simulink model "TST_AFST_DD"  (R2016b)
settings: Solver=FixedStepDiscrete  StartTime=0.0  StopTime=simTime  FixedStep=sampleTime  RelTol=1e-3
values from neighbouring files (symbols this model uses):
  testCase = 1    [initTST_AFST_DD_001.m]    (also in initTST_AFST_DD_002.m = 2; initTST_AFST_DD_003.m = 3; initTST_AFST_DD_004.m = 4)
libraries: simulink x61, UnitTest_Lib x56
(part 2 of 2)

== system TST_AFST_DD/simulationInput/testSignals_R004 ==
  BC : BusCreator  Inputs=19
  spec_Air_bDtyCycHiDebTAFS_DSM : FromWorkspace  VariableName=testSig_Air_bDtyCycHiDebTAFS_DSM  Interpolate=off  OutputAfterFinalValue=Holding final value
  spec_Air_bDtyCycLoDebTAFS_DSM : FromWorkspace  VariableName=testSig_Air_bDtyCycLoDebTAFS_DSM  Interpolate=off  OutputAfterFinalValue=Holding final value
  spec_Air_bDtyCycTAFSFinalDef : FromWorkspace  VariableName=testSig_Air_bDtyCycTAFSFinalDef  Interpolate=off  OutputAfterFinalValue=Holding final value
  spec_Air_bDtyCycTAFSProvDef : FromWorkspace  VariableName=testSig_Air_bDtyCycTAFSProvDef  Interpolate=off  OutputAfterFinalValue=Holding final value
  spec_Air_bPerHiDebTAFS_DSM : FromWorkspace  VariableName=testSig_Air_bPerHiDebTAFS_DSM  Interpolate=off  OutputAfterFinalValue=Holding final value
  spec_Air_bPerLoDebTAFS_DSM : FromWorkspace  VariableName=testSig_Air_bPerLoDebTAFS_DSM  Interpolate=off  OutputAfterFinalValue=Holding final value
  spec_Air_bPerTAFSFinalDef : FromWorkspace  VariableName=testSig_Air_bPerTAFSFinalDef  Interpolate=off  OutputAfterFinalValue=Holding final value
  spec_Air_bPerTAFSProvDef : FromWorkspace  VariableName=testSig_Air_bPerTAFSProvDef  Interpolate=off  OutputAfterFinalValue=Holding final value
  spec_Air_bVoltHiDebTAFS_DSM : FromWorkspace  VariableName=testSig_Air_bVoltHiDebTAFS_DSM  Interpolate=off  OutputAfterFinalValue=Holding final value
  spec_Air_bVoltLoDebTAFS_DSM : FromWorkspace  VariableName=testSig_Air_bVoltLoDebTAFS_DSM  Interpolate=off  OutputAfterFinalValue=Holding final value
  spec_Air_bVoltTAFSFinalDef : FromWorkspace  VariableName=testSig_Air_bVoltTAFSFinalDef  Interpolate=off  OutputAfterFinalValue=Holding final value
  spec_Air_bVoltTAFSProvDef : FromWorkspace  VariableName=testSig_Air_bVoltTAFSProvDef  Interpolate=off  OutputAfterFinalValue=Holding final value
  spec_Air_facPerCorTAFS : FromWorkspace  VariableName=testSig_Air_facPerCorTAFS  Interpolate=off  OutputAfterFinalValue=Holding final value
  spec_Air_rRawTAFS : FromWorkspace  VariableName=testSig_Air_rRawTAFS  Interpolate=off  OutputAfterFinalValue=Holding final value
  spec_Air_tSensTAFS : FromWorkspace  VariableName=testSig_Air_tSensTAFS  Interpolate=off  OutputAfterFinalValue=Holding final value
  spec_Air_tiRawTAFS : FromWorkspace  VariableName=testSig_Air_tiRawTAFS  Interpolate=off  OutputAfterFinalValue=Holding final value
  spec_Air_uRawTAFS : FromWorkspace  VariableName=testSig_Air_uRawTAFS  Interpolate=off  OutputAfterFinalValue=Holding final value
  spec_DSM_bTAFSSigMonRls : FromWorkspace  VariableName=testSig_DSM_bTAFSSigMonRls  Interpolate=off  OutputAfterFinalValue=Holding final value
  spec_T15_st : FromWorkspace  VariableName=testSig_T15_st  Interpolate=off  OutputAfterFinalValue=Holding final value
  testSignals : Outport
  wires:
  BC/1 -> testSignals/1
  spec_T15_st/1 -> BC/1  "testSig_T15_st"
  spec_Air_rRawTAFS/1 -> BC/2  "testSig_Air_rRawTAFS"
  spec_Air_tiRawTAFS/1 -> BC/3  "testSig_Air_tiRawTAFS"
  spec_DSM_bTAFSSigMonRls/1 -> BC/4  "testSig_DSM_bTAFSSigMonRls"
  spec_Air_uRawTAFS/1 -> BC/5  "testSig_Air_uRawTAFS"
  spec_Air_tSensTAFS/1 -> BC/6  "testSig_Air_tSensTAFS"
  spec_Air_bDtyCycTAFSFinalDef/1 -> BC/7  "testSig_Air_bDtyCycTAFSFinalDef"
  spec_Air_bDtyCycTAFSProvDef/1 -> BC/8  "testSig_Air_bDtyCycTAFSProvDef"
  spec_Air_bPerTAFSFinalDef/1 -> BC/9  "testSig_Air_bPerTAFSFinalDef"
  spec_Air_bPerTAFSProvDef/1 -> BC/10  "testSig_Air_bPerTAFSProvDef"
  spec_Air_facPerCorTAFS/1 -> BC/11  "testSig_Air_facPerCorTAFS"
  spec_Air_bDtyCycHiDebTAFS_DSM/1 -> BC/12  "testSig_Air_bDtyCycHiDebTAFS_DSM"
  spec_Air_bDtyCycLoDebTAFS_DSM/1 -> BC/13  "testSig_Air_bDtyCycLoDebTAFS_DSM"
  spec_Air_bPerHiDebTAFS_DSM/1 -> BC/14  "testSig_Air_bPerHiDebTAFS_DSM"
  spec_Air_bPerLoDebTAFS_DSM/1 -> BC/15  "testSig_Air_bPerLoDebTAFS_DSM"
  spec_Air_bVoltTAFSFinalDef/1 -> BC/16  "testSig_Air_bVoltTAFSFinalDef"
  spec_Air_bVoltTAFSProvDef/1 -> BC/17  "testSig_Air_bVoltTAFSProvDef"
  spec_Air_bVoltHiDebTAFS_DSM/1 -> BC/18  "testSig_Air_bVoltHiDebTAFS_DSM"
  spec_Air_bVoltLoDebTAFS_DSM/1 -> BC/19  "testSig_Air_bVoltLoDebTAFS_DSM"

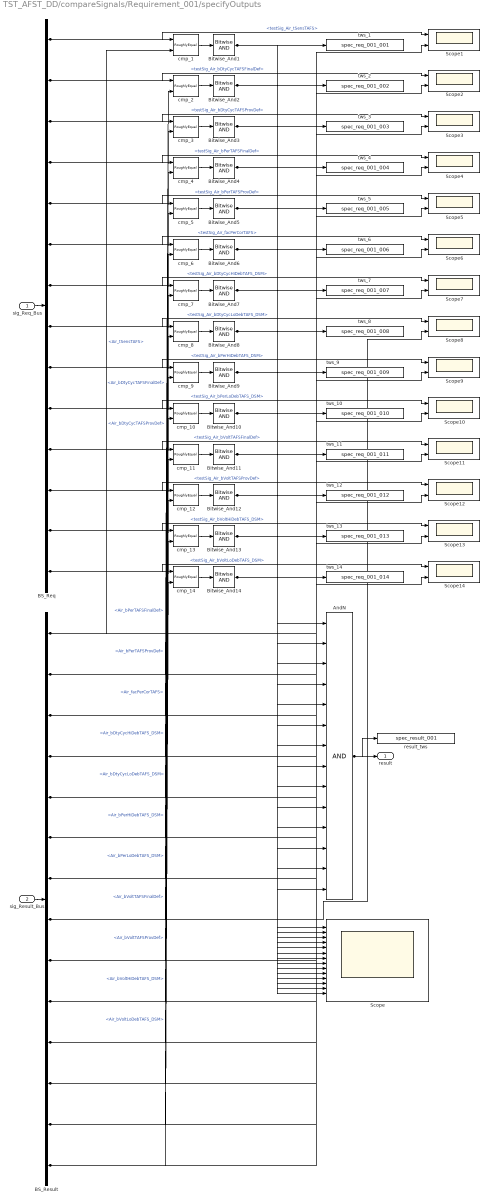
== system TST_AFST_DD/compareSignals/Requirement_001/specifyOutputs ==
  sig_Req_Bus : Inport
  sig_Result_Bus : Inport  Port=2
  AndN : Logic  Inputs=14
  BS_Req : BusSelector  OutputSignals=testSig_Air_tSensTAFS,testSig_Air_bDtyCycTAFSFinalDef,testSig_Air_bDtyCycTAFSProvDef,testSig_Air_bPerTAFSFinalDef,testSig_Air_bPerTAFSProvDef,testSig_Air_facPerCorTAFS,testSig_Air_bDtyCycHiDebTAFS_DSM,testSig_Air_bDtyCycLoDebTAFS_DSM,testSig_Air_bPerHiDebTAFS_DSM,testSig_Air_bPerLoDebTAFS_DSM,testSig_Air_bVoltTAFSFinalDef,testSig_Air_bVoltTAFSProvDef,testSig_Air_bVoltHiDebTAFS_DSM,testSig_Air_bVoltLoDebTAFS_DSM
  BS_Result : BusSelector  OutputSignals=Air_tSensTAFS,Air_bDtyCycTAFSFinalDef,Air_bDtyCycTAFSProvDef,Air_bPerTAFSFinalDef,Air_bPerTAFSProvDef,Air_facPerCorTAFS,Air_bDtyCycHiDebTAFS_DSM,Air_bDtyCycLoDebTAFS_DSM,Air_bPerHiDebTAFS_DSM,Air_bPerLoDebTAFS_DSM,Air_bVoltTAFSFinalDef,Air_bVoltTAFSProvDef,Air_bVoltHiDebTAFS_DSM,Air_bVoltLoDebTAFS_DSM
  Bitwise_And{1..14} (14 alike) : simulink/Logic and Bit Operations/Bitwise Operator  logicop=AND  UseBitMask=off  BitMask=bin2dec('11011001')  BitMaskRealWorld=Stored Integer
  Scope : Scope  NumInputPorts=14
  Scope{1..14} (14 alike) : Scope  NumInputPorts=2
  cmp_{1..14} (14 alike) : UnitTest_Lib/RoughlyEqual  slope=0.1
  result_tws : ToWorkspace  VariableName=spec_result_001
  tws_1 : ToWorkspace  VariableName=spec_req_001_001
  tws_10 : ToWorkspace  VariableName=spec_req_001_010
  tws_11 : ToWorkspace  VariableName=spec_req_001_011
  tws_12 : ToWorkspace  VariableName=spec_req_001_012
  tws_13 : ToWorkspace  VariableName=spec_req_001_013
  tws_14 : ToWorkspace  VariableName=spec_req_001_014
  tws_2 : ToWorkspace  VariableName=spec_req_001_002
  tws_3 : ToWorkspace  VariableName=spec_req_001_003
  tws_4 : ToWorkspace  VariableName=spec_req_001_004
  tws_5 : ToWorkspace  VariableName=spec_req_001_005
  tws_6 : ToWorkspace  VariableName=spec_req_001_006
  tws_7 : ToWorkspace  VariableName=spec_req_001_007
  tws_8 : ToWorkspace  VariableName=spec_req_001_008
  tws_9 : ToWorkspace  VariableName=spec_req_001_009
  result : Outport
  wires:
  sig_Req_Bus/1 -> BS_Req/1
  sig_Result_Bus/1 -> BS_Result/1
  AndN/1 -> result/1, result_tws/1
  BS_Req/1 -> cmp_1/1, Scope1/1  "<testSig_Air_tSensTAFS>"
  BS_Result/1 -> cmp_1/2, Scope1/2  "<Air_tSensTAFS>"
  cmp_1/1 -> Bitwise_And1/1
  Bitwise_And1/1 -> tws_1/1, AndN/1, Scope/1
  BS_Req/2 -> cmp_2/1, Scope2/1  "<testSig_Air_bDtyCycTAFSFinalDef>"
  BS_Result/2 -> cmp_2/2, Scope2/2  "<Air_bDtyCycTAFSFinalDef>"
  cmp_2/1 -> Bitwise_And2/1
  Bitwise_And2/1 -> tws_2/1, AndN/2, Scope/2
  BS_Req/3 -> cmp_3/1, Scope3/1  "<testSig_Air_bDtyCycTAFSProvDef>"
  BS_Result/3 -> cmp_3/2, Scope3/2  "<Air_bDtyCycTAFSProvDef>"
  cmp_3/1 -> Bitwise_And3/1
  Bitwise_And3/1 -> tws_3/1, AndN/3, Scope/3
  BS_Req/4 -> cmp_4/1, Scope4/1  "<testSig_Air_bPerTAFSFinalDef>"
  BS_Result/4 -> cmp_4/2, Scope4/2  "<Air_bPerTAFSFinalDef>"
  cmp_4/1 -> Bitwise_And4/1
  Bitwise_And4/1 -> tws_4/1, AndN/4, Scope/4
  BS_Req/5 -> cmp_5/1, Scope5/1  "<testSig_Air_bPerTAFSProvDef>"
  BS_Result/5 -> cmp_5/2, Scope5/2  "<Air_bPerTAFSProvDef>"
  cmp_5/1 -> Bitwise_And5/1
  Bitwise_And5/1 -> tws_5/1, AndN/5, Scope/5
  BS_Req/6 -> cmp_6/1, Scope6/1  "<testSig_Air_facPerCorTAFS>"
  BS_Result/6 -> cmp_6/2, Scope6/2  "<Air_facPerCorTAFS>"
  cmp_6/1 -> Bitwise_And6/1
  Bitwise_And6/1 -> tws_6/1, AndN/6, Scope/6
  BS_Req/7 -> cmp_7/1, Scope7/1  "<testSig_Air_bDtyCycHiDebTAFS_DSM>"
  BS_Result/7 -> cmp_7/2, Scope7/2  "<Air_bDtyCycHiDebTAFS_DSM>"
  cmp_7/1 -> Bitwise_And7/1
  Bitwise_And7/1 -> tws_7/1, AndN/7, Scope/7
  BS_Req/8 -> cmp_8/1, Scope8/1  "<testSig_Air_bDtyCycLoDebTAFS_DSM>"
  BS_Result/8 -> cmp_8/2, Scope8/2  "<Air_bDtyCycLoDebTAFS_DSM>"
  cmp_8/1 -> Bitwise_And8/1
  Bitwise_And8/1 -> tws_8/1, AndN/8, Scope/8
  BS_Req/9 -> cmp_9/1, Scope9/1  "<testSig_Air_bPerHiDebTAFS_DSM>"
  BS_Result/9 -> cmp_9/2, Scope9/2  "<Air_bPerHiDebTAFS_DSM>"
  cmp_9/1 -> Bitwise_And9/1
  Bitwise_And9/1 -> tws_9/1, AndN/9, Scope/9
  BS_Req/10 -> cmp_10/1, Scope10/1  "<testSig_Air_bPerLoDebTAFS_DSM>"
  BS_Result/10 -> cmp_10/2, Scope10/2  "<Air_bPerLoDebTAFS_DSM>"
  cmp_10/1 -> Bitwise_And10/1
  Bitwise_And10/1 -> tws_10/1, AndN/10, Scope/10
  BS_Req/11 -> cmp_11/1, Scope11/1  "<testSig_Air_bVoltTAFSFinalDef>"
  BS_Result/11 -> cmp_11/2, Scope11/2  "<Air_bVoltTAFSFinalDef>"
  cmp_11/1 -> Bitwise_And11/1
  Bitwise_And11/1 -> tws_11/1, AndN/11, Scope/11
  BS_Req/12 -> cmp_12/1, Scope12/1  "<testSig_Air_bVoltTAFSProvDef>"
  BS_Result/12 -> cmp_12/2, Scope12/2  "<Air_bVoltTAFSProvDef>"
  cmp_12/1 -> Bitwise_And12/1
  Bitwise_And12/1 -> tws_12/1, AndN/12, Scope/12
  BS_Req/13 -> cmp_13/1, Scope13/1  "<testSig_Air_bVoltHiDebTAFS_DSM>"
  BS_Result/13 -> cmp_13/2, Scope13/2  "<Air_bVoltHiDebTAFS_DSM>"
  cmp_13/1 -> Bitwise_And13/1
  Bitwise_And13/1 -> tws_13/1, AndN/13, Scope/13
  BS_Req/14 -> cmp_14/1, Scope14/1  "<testSig_Air_bVoltLoDebTAFS_DSM>"
  BS_Result/14 -> cmp_14/2, Scope14/2  "<Air_bVoltLoDebTAFS_DSM>"
  cmp_14/1 -> Bitwise_And14/1
  Bitwise_And14/1 -> tws_14/1, AndN/14, Scope/14

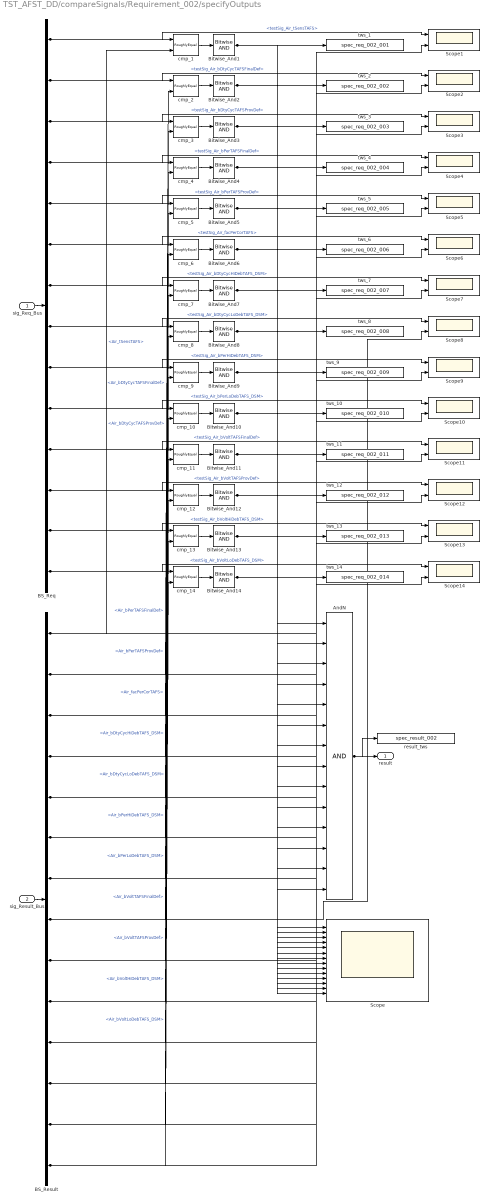
== system TST_AFST_DD/compareSignals/Requirement_002/specifyOutputs ==
  sig_Req_Bus : Inport
  sig_Result_Bus : Inport  Port=2
  AndN : Logic  Inputs=14
  BS_Req : BusSelector  OutputSignals=testSig_Air_tSensTAFS,testSig_Air_bDtyCycTAFSFinalDef,testSig_Air_bDtyCycTAFSProvDef,testSig_Air_bPerTAFSFinalDef,testSig_Air_bPerTAFSProvDef,testSig_Air_facPerCorTAFS,testSig_Air_bDtyCycHiDebTAFS_DSM,testSig_Air_bDtyCycLoDebTAFS_DSM,testSig_Air_bPerHiDebTAFS_DSM,testSig_Air_bPerLoDebTAFS_DSM,testSig_Air_bVoltTAFSFinalDef,testSig_Air_bVoltTAFSProvDef,testSig_Air_bVoltHiDebTAFS_DSM,testSig_Air_bVoltLoDebTAFS_DSM
  BS_Result : BusSelector  OutputSignals=Air_tSensTAFS,Air_bDtyCycTAFSFinalDef,Air_bDtyCycTAFSProvDef,Air_bPerTAFSFinalDef,Air_bPerTAFSProvDef,Air_facPerCorTAFS,Air_bDtyCycHiDebTAFS_DSM,Air_bDtyCycLoDebTAFS_DSM,Air_bPerHiDebTAFS_DSM,Air_bPerLoDebTAFS_DSM,Air_bVoltTAFSFinalDef,Air_bVoltTAFSProvDef,Air_bVoltHiDebTAFS_DSM,Air_bVoltLoDebTAFS_DSM
  Bitwise_And{1..14} (14 alike) : simulink/Logic and Bit Operations/Bitwise Operator  logicop=AND  UseBitMask=off  BitMask=bin2dec('11011001')  BitMaskRealWorld=Stored Integer
  Scope : Scope  NumInputPorts=14
  Scope{1..14} (14 alike) : Scope  NumInputPorts=2
  cmp_{1..14} (14 alike) : UnitTest_Lib/RoughlyEqual  slope=0.1
  result_tws : ToWorkspace  VariableName=spec_result_002
  tws_1 : ToWorkspace  VariableName=spec_req_002_001
  tws_10 : ToWorkspace  VariableName=spec_req_002_010
  tws_11 : ToWorkspace  VariableName=spec_req_002_011
  tws_12 : ToWorkspace  VariableName=spec_req_002_012
  tws_13 : ToWorkspace  VariableName=spec_req_002_013
  tws_14 : ToWorkspace  VariableName=spec_req_002_014
  tws_2 : ToWorkspace  VariableName=spec_req_002_002
  tws_3 : ToWorkspace  VariableName=spec_req_002_003
  tws_4 : ToWorkspace  VariableName=spec_req_002_004
  tws_5 : ToWorkspace  VariableName=spec_req_002_005
  tws_6 : ToWorkspace  VariableName=spec_req_002_006
  tws_7 : ToWorkspace  VariableName=spec_req_002_007
  tws_8 : ToWorkspace  VariableName=spec_req_002_008
  tws_9 : ToWorkspace  VariableName=spec_req_002_009
  result : Outport
  wires:
  sig_Req_Bus/1 -> BS_Req/1
  sig_Result_Bus/1 -> BS_Result/1
  AndN/1 -> result/1, result_tws/1
  BS_Req/1 -> cmp_1/1, Scope1/1  "<testSig_Air_tSensTAFS>"
  BS_Result/1 -> cmp_1/2, Scope1/2  "<Air_tSensTAFS>"
  cmp_1/1 -> Bitwise_And1/1
  Bitwise_And1/1 -> tws_1/1, AndN/1, Scope/1
  BS_Req/2 -> cmp_2/1, Scope2/1  "<testSig_Air_bDtyCycTAFSFinalDef>"
  BS_Result/2 -> cmp_2/2, Scope2/2  "<Air_bDtyCycTAFSFinalDef>"
  cmp_2/1 -> Bitwise_And2/1
  Bitwise_And2/1 -> tws_2/1, AndN/2, Scope/2
  BS_Req/3 -> cmp_3/1, Scope3/1  "<testSig_Air_bDtyCycTAFSProvDef>"
  BS_Result/3 -> cmp_3/2, Scope3/2  "<Air_bDtyCycTAFSProvDef>"
  cmp_3/1 -> Bitwise_And3/1
  Bitwise_And3/1 -> tws_3/1, AndN/3, Scope/3
  BS_Req/4 -> cmp_4/1, Scope4/1  "<testSig_Air_bPerTAFSFinalDef>"
  BS_Result/4 -> cmp_4/2, Scope4/2  "<Air_bPerTAFSFinalDef>"
  cmp_4/1 -> Bitwise_And4/1
  Bitwise_And4/1 -> tws_4/1, AndN/4, Scope/4
  BS_Req/5 -> cmp_5/1, Scope5/1  "<testSig_Air_bPerTAFSProvDef>"
  BS_Result/5 -> cmp_5/2, Scope5/2  "<Air_bPerTAFSProvDef>"
  cmp_5/1 -> Bitwise_And5/1
  Bitwise_And5/1 -> tws_5/1, AndN/5, Scope/5
  BS_Req/6 -> cmp_6/1, Scope6/1  "<testSig_Air_facPerCorTAFS>"
  BS_Result/6 -> cmp_6/2, Scope6/2  "<Air_facPerCorTAFS>"
  cmp_6/1 -> Bitwise_And6/1
  Bitwise_And6/1 -> tws_6/1, AndN/6, Scope/6
  BS_Req/7 -> cmp_7/1, Scope7/1  "<testSig_Air_bDtyCycHiDebTAFS_DSM>"
  BS_Result/7 -> cmp_7/2, Scope7/2  "<Air_bDtyCycHiDebTAFS_DSM>"
  cmp_7/1 -> Bitwise_And7/1
  Bitwise_And7/1 -> tws_7/1, AndN/7, Scope/7
  BS_Req/8 -> cmp_8/1, Scope8/1  "<testSig_Air_bDtyCycLoDebTAFS_DSM>"
  BS_Result/8 -> cmp_8/2, Scope8/2  "<Air_bDtyCycLoDebTAFS_DSM>"
  cmp_8/1 -> Bitwise_And8/1
  Bitwise_And8/1 -> tws_8/1, AndN/8, Scope/8
  BS_Req/9 -> cmp_9/1, Scope9/1  "<testSig_Air_bPerHiDebTAFS_DSM>"
  BS_Result/9 -> cmp_9/2, Scope9/2  "<Air_bPerHiDebTAFS_DSM>"
  cmp_9/1 -> Bitwise_And9/1
  Bitwise_And9/1 -> tws_9/1, AndN/9, Scope/9
  BS_Req/10 -> cmp_10/1, Scope10/1  "<testSig_Air_bPerLoDebTAFS_DSM>"
  BS_Result/10 -> cmp_10/2, Scope10/2  "<Air_bPerLoDebTAFS_DSM>"
  cmp_10/1 -> Bitwise_And10/1
  Bitwise_And10/1 -> tws_10/1, AndN/10, Scope/10
  BS_Req/11 -> cmp_11/1, Scope11/1  "<testSig_Air_bVoltTAFSFinalDef>"
  BS_Result/11 -> cmp_11/2, Scope11/2  "<Air_bVoltTAFSFinalDef>"
  cmp_11/1 -> Bitwise_And11/1
  Bitwise_And11/1 -> tws_11/1, AndN/11, Scope/11
  BS_Req/12 -> cmp_12/1, Scope12/1  "<testSig_Air_bVoltTAFSProvDef>"
  BS_Result/12 -> cmp_12/2, Scope12/2  "<Air_bVoltTAFSProvDef>"
  cmp_12/1 -> Bitwise_And12/1
  Bitwise_And12/1 -> tws_12/1, AndN/12, Scope/12
  BS_Req/13 -> cmp_13/1, Scope13/1  "<testSig_Air_bVoltHiDebTAFS_DSM>"
  BS_Result/13 -> cmp_13/2, Scope13/2  "<Air_bVoltHiDebTAFS_DSM>"
  cmp_13/1 -> Bitwise_And13/1
  Bitwise_And13/1 -> tws_13/1, AndN/13, Scope/13
  BS_Req/14 -> cmp_14/1, Scope14/1  "<testSig_Air_bVoltLoDebTAFS_DSM>"
  BS_Result/14 -> cmp_14/2, Scope14/2  "<Air_bVoltLoDebTAFS_DSM>"
  cmp_14/1 -> Bitwise_And14/1
  Bitwise_And14/1 -> tws_14/1, AndN/14, Scope/14

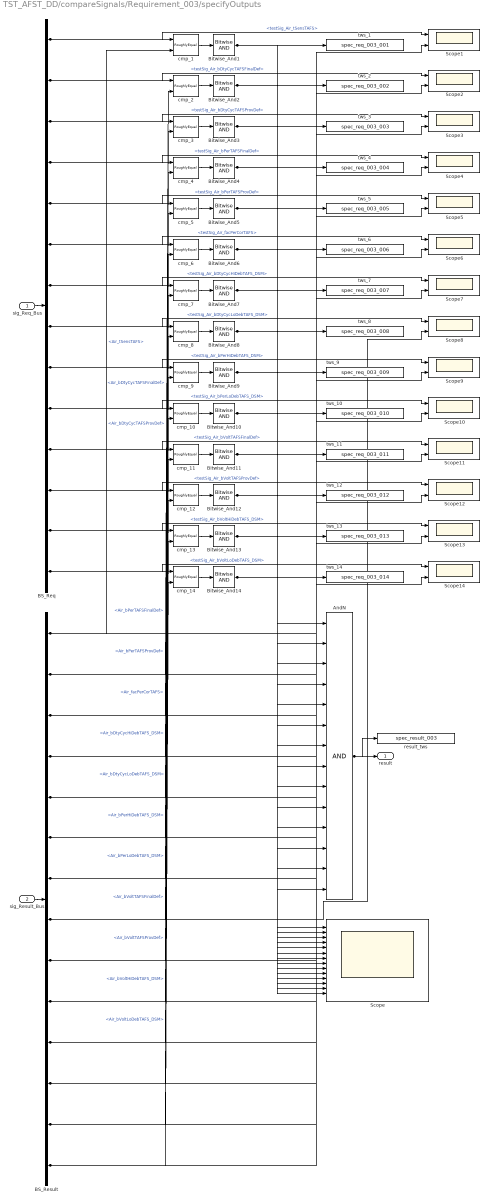
== system TST_AFST_DD/compareSignals/Requirement_003/specifyOutputs ==
  sig_Req_Bus : Inport
  sig_Result_Bus : Inport  Port=2
  AndN : Logic  Inputs=14
  BS_Req : BusSelector  OutputSignals=testSig_Air_tSensTAFS,testSig_Air_bDtyCycTAFSFinalDef,testSig_Air_bDtyCycTAFSProvDef,testSig_Air_bPerTAFSFinalDef,testSig_Air_bPerTAFSProvDef,testSig_Air_facPerCorTAFS,testSig_Air_bDtyCycHiDebTAFS_DSM,testSig_Air_bDtyCycLoDebTAFS_DSM,testSig_Air_bPerHiDebTAFS_DSM,testSig_Air_bPerLoDebTAFS_DSM,testSig_Air_bVoltTAFSFinalDef,testSig_Air_bVoltTAFSProvDef,testSig_Air_bVoltHiDebTAFS_DSM,testSig_Air_bVoltLoDebTAFS_DSM
  BS_Result : BusSelector  OutputSignals=Air_tSensTAFS,Air_bDtyCycTAFSFinalDef,Air_bDtyCycTAFSProvDef,Air_bPerTAFSFinalDef,Air_bPerTAFSProvDef,Air_facPerCorTAFS,Air_bDtyCycHiDebTAFS_DSM,Air_bDtyCycLoDebTAFS_DSM,Air_bPerHiDebTAFS_DSM,Air_bPerLoDebTAFS_DSM,Air_bVoltTAFSFinalDef,Air_bVoltTAFSProvDef,Air_bVoltHiDebTAFS_DSM,Air_bVoltLoDebTAFS_DSM
  Bitwise_And{1..14} (14 alike) : simulink/Logic and Bit Operations/Bitwise Operator  logicop=AND  UseBitMask=off  BitMask=bin2dec('11011001')  BitMaskRealWorld=Stored Integer
  Scope : Scope  NumInputPorts=14
  Scope{1..14} (14 alike) : Scope  NumInputPorts=2
  cmp_{1..14} (14 alike) : UnitTest_Lib/RoughlyEqual  slope=0.1
  result_tws : ToWorkspace  VariableName=spec_result_003
  tws_1 : ToWorkspace  VariableName=spec_req_003_001
  tws_10 : ToWorkspace  VariableName=spec_req_003_010
  tws_11 : ToWorkspace  VariableName=spec_req_003_011
  tws_12 : ToWorkspace  VariableName=spec_req_003_012
  tws_13 : ToWorkspace  VariableName=spec_req_003_013
  tws_14 : ToWorkspace  VariableName=spec_req_003_014
  tws_2 : ToWorkspace  VariableName=spec_req_003_002
  tws_3 : ToWorkspace  VariableName=spec_req_003_003
  tws_4 : ToWorkspace  VariableName=spec_req_003_004
  tws_5 : ToWorkspace  VariableName=spec_req_003_005
  tws_6 : ToWorkspace  VariableName=spec_req_003_006
  tws_7 : ToWorkspace  VariableName=spec_req_003_007
  tws_8 : ToWorkspace  VariableName=spec_req_003_008
  tws_9 : ToWorkspace  VariableName=spec_req_003_009
  result : Outport
  wires:
  sig_Req_Bus/1 -> BS_Req/1
  sig_Result_Bus/1 -> BS_Result/1
  AndN/1 -> result/1, result_tws/1
  BS_Req/1 -> cmp_1/1, Scope1/1  "<testSig_Air_tSensTAFS>"
  BS_Result/1 -> cmp_1/2, Scope1/2  "<Air_tSensTAFS>"
  cmp_1/1 -> Bitwise_And1/1
  Bitwise_And1/1 -> tws_1/1, AndN/1, Scope/1
  BS_Req/2 -> cmp_2/1, Scope2/1  "<testSig_Air_bDtyCycTAFSFinalDef>"
  BS_Result/2 -> cmp_2/2, Scope2/2  "<Air_bDtyCycTAFSFinalDef>"
  cmp_2/1 -> Bitwise_And2/1
  Bitwise_And2/1 -> tws_2/1, AndN/2, Scope/2
  BS_Req/3 -> cmp_3/1, Scope3/1  "<testSig_Air_bDtyCycTAFSProvDef>"
  BS_Result/3 -> cmp_3/2, Scope3/2  "<Air_bDtyCycTAFSProvDef>"
  cmp_3/1 -> Bitwise_And3/1
  Bitwise_And3/1 -> tws_3/1, AndN/3, Scope/3
  BS_Req/4 -> cmp_4/1, Scope4/1  "<testSig_Air_bPerTAFSFinalDef>"
  BS_Result/4 -> cmp_4/2, Scope4/2  "<Air_bPerTAFSFinalDef>"
  cmp_4/1 -> Bitwise_And4/1
  Bitwise_And4/1 -> tws_4/1, AndN/4, Scope/4
  BS_Req/5 -> cmp_5/1, Scope5/1  "<testSig_Air_bPerTAFSProvDef>"
  BS_Result/5 -> cmp_5/2, Scope5/2  "<Air_bPerTAFSProvDef>"
  cmp_5/1 -> Bitwise_And5/1
  Bitwise_And5/1 -> tws_5/1, AndN/5, Scope/5
  BS_Req/6 -> cmp_6/1, Scope6/1  "<testSig_Air_facPerCorTAFS>"
  BS_Result/6 -> cmp_6/2, Scope6/2  "<Air_facPerCorTAFS>"
  cmp_6/1 -> Bitwise_And6/1
  Bitwise_And6/1 -> tws_6/1, AndN/6, Scope/6
  BS_Req/7 -> cmp_7/1, Scope7/1  "<testSig_Air_bDtyCycHiDebTAFS_DSM>"
  BS_Result/7 -> cmp_7/2, Scope7/2  "<Air_bDtyCycHiDebTAFS_DSM>"
  cmp_7/1 -> Bitwise_And7/1
  Bitwise_And7/1 -> tws_7/1, AndN/7, Scope/7
  BS_Req/8 -> cmp_8/1, Scope8/1  "<testSig_Air_bDtyCycLoDebTAFS_DSM>"
  BS_Result/8 -> cmp_8/2, Scope8/2  "<Air_bDtyCycLoDebTAFS_DSM>"
  cmp_8/1 -> Bitwise_And8/1
  Bitwise_And8/1 -> tws_8/1, AndN/8, Scope/8
  BS_Req/9 -> cmp_9/1, Scope9/1  "<testSig_Air_bPerHiDebTAFS_DSM>"
  BS_Result/9 -> cmp_9/2, Scope9/2  "<Air_bPerHiDebTAFS_DSM>"
  cmp_9/1 -> Bitwise_And9/1
  Bitwise_And9/1 -> tws_9/1, AndN/9, Scope/9
  BS_Req/10 -> cmp_10/1, Scope10/1  "<testSig_Air_bPerLoDebTAFS_DSM>"
  BS_Result/10 -> cmp_10/2, Scope10/2  "<Air_bPerLoDebTAFS_DSM>"
  cmp_10/1 -> Bitwise_And10/1
  Bitwise_And10/1 -> tws_10/1, AndN/10, Scope/10
  BS_Req/11 -> cmp_11/1, Scope11/1  "<testSig_Air_bVoltTAFSFinalDef>"
  BS_Result/11 -> cmp_11/2, Scope11/2  "<Air_bVoltTAFSFinalDef>"
  cmp_11/1 -> Bitwise_And11/1
  Bitwise_And11/1 -> tws_11/1, AndN/11, Scope/11
  BS_Req/12 -> cmp_12/1, Scope12/1  "<testSig_Air_bVoltTAFSProvDef>"
  BS_Result/12 -> cmp_12/2, Scope12/2  "<Air_bVoltTAFSProvDef>"
  cmp_12/1 -> Bitwise_And12/1
  Bitwise_And12/1 -> tws_12/1, AndN/12, Scope/12
  BS_Req/13 -> cmp_13/1, Scope13/1  "<testSig_Air_bVoltHiDebTAFS_DSM>"
  BS_Result/13 -> cmp_13/2, Scope13/2  "<Air_bVoltHiDebTAFS_DSM>"
  cmp_13/1 -> Bitwise_And13/1
  Bitwise_And13/1 -> tws_13/1, AndN/13, Scope/13
  BS_Req/14 -> cmp_14/1, Scope14/1  "<testSig_Air_bVoltLoDebTAFS_DSM>"
  BS_Result/14 -> cmp_14/2, Scope14/2  "<Air_bVoltLoDebTAFS_DSM>"
  cmp_14/1 -> Bitwise_And14/1
  Bitwise_And14/1 -> tws_14/1, AndN/14, Scope/14

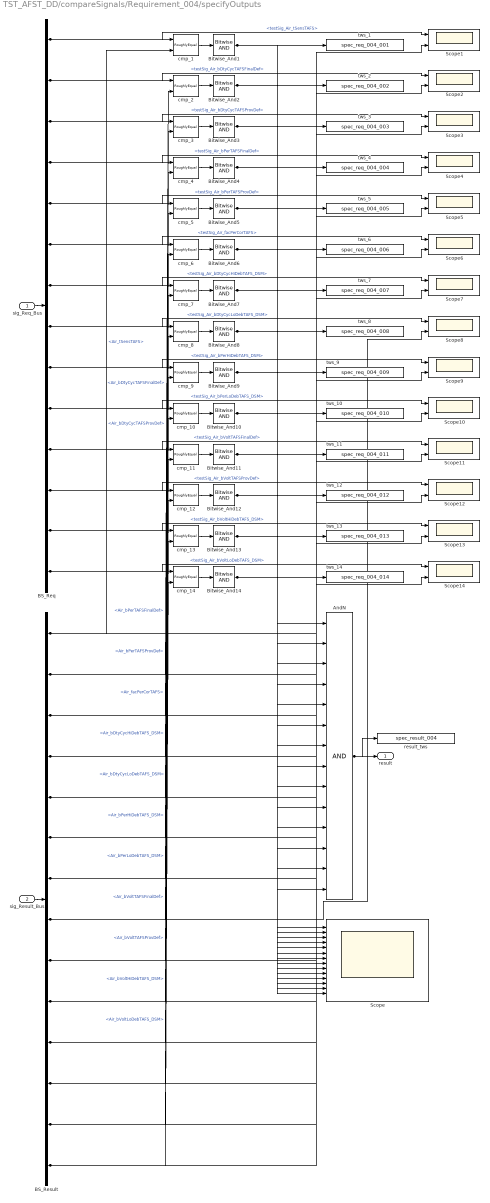
== system TST_AFST_DD/compareSignals/Requirement_004/specifyOutputs ==
  sig_Req_Bus : Inport
  sig_Result_Bus : Inport  Port=2
  AndN : Logic  Inputs=14
  BS_Req : BusSelector  OutputSignals=testSig_Air_tSensTAFS,testSig_Air_bDtyCycTAFSFinalDef,testSig_Air_bDtyCycTAFSProvDef,testSig_Air_bPerTAFSFinalDef,testSig_Air_bPerTAFSProvDef,testSig_Air_facPerCorTAFS,testSig_Air_bDtyCycHiDebTAFS_DSM,testSig_Air_bDtyCycLoDebTAFS_DSM,testSig_Air_bPerHiDebTAFS_DSM,testSig_Air_bPerLoDebTAFS_DSM,testSig_Air_bVoltTAFSFinalDef,testSig_Air_bVoltTAFSProvDef,testSig_Air_bVoltHiDebTAFS_DSM,testSig_Air_bVoltLoDebTAFS_DSM
  BS_Result : BusSelector  OutputSignals=Air_tSensTAFS,Air_bDtyCycTAFSFinalDef,Air_bDtyCycTAFSProvDef,Air_bPerTAFSFinalDef,Air_bPerTAFSProvDef,Air_facPerCorTAFS,Air_bDtyCycHiDebTAFS_DSM,Air_bDtyCycLoDebTAFS_DSM,Air_bPerHiDebTAFS_DSM,Air_bPerLoDebTAFS_DSM,Air_bVoltTAFSFinalDef,Air_bVoltTAFSProvDef,Air_bVoltHiDebTAFS_DSM,Air_bVoltLoDebTAFS_DSM
  Bitwise_And{1..14} (14 alike) : simulink/Logic and Bit Operations/Bitwise Operator  logicop=AND  UseBitMask=off  BitMask=bin2dec('11011001')  BitMaskRealWorld=Stored Integer
  Scope : Scope  NumInputPorts=14
  Scope{1..14} (14 alike) : Scope  NumInputPorts=2
  cmp_{1..14} (14 alike) : UnitTest_Lib/RoughlyEqual  slope=0.1
  result_tws : ToWorkspace  VariableName=spec_result_004
  tws_1 : ToWorkspace  VariableName=spec_req_004_001
  tws_10 : ToWorkspace  VariableName=spec_req_004_010
  tws_11 : ToWorkspace  VariableName=spec_req_004_011
  tws_12 : ToWorkspace  VariableName=spec_req_004_012
  tws_13 : ToWorkspace  VariableName=spec_req_004_013
  tws_14 : ToWorkspace  VariableName=spec_req_004_014
  tws_2 : ToWorkspace  VariableName=spec_req_004_002
  tws_3 : ToWorkspace  VariableName=spec_req_004_003
  tws_4 : ToWorkspace  VariableName=spec_req_004_004
  tws_5 : ToWorkspace  VariableName=spec_req_004_005
  tws_6 : ToWorkspace  VariableName=spec_req_004_006
  tws_7 : ToWorkspace  VariableName=spec_req_004_007
  tws_8 : ToWorkspace  VariableName=spec_req_004_008
  tws_9 : ToWorkspace  VariableName=spec_req_004_009
  result : Outport
  wires:
  sig_Req_Bus/1 -> BS_Req/1
  sig_Result_Bus/1 -> BS_Result/1
  AndN/1 -> result/1, result_tws/1
  BS_Req/1 -> cmp_1/1, Scope1/1  "<testSig_Air_tSensTAFS>"
  BS_Result/1 -> cmp_1/2, Scope1/2  "<Air_tSensTAFS>"
  cmp_1/1 -> Bitwise_And1/1
  Bitwise_And1/1 -> tws_1/1, AndN/1, Scope/1
  BS_Req/2 -> cmp_2/1, Scope2/1  "<testSig_Air_bDtyCycTAFSFinalDef>"
  BS_Result/2 -> cmp_2/2, Scope2/2  "<Air_bDtyCycTAFSFinalDef>"
  cmp_2/1 -> Bitwise_And2/1
  Bitwise_And2/1 -> tws_2/1, AndN/2, Scope/2
  BS_Req/3 -> cmp_3/1, Scope3/1  "<testSig_Air_bDtyCycTAFSProvDef>"
  BS_Result/3 -> cmp_3/2, Scope3/2  "<Air_bDtyCycTAFSProvDef>"
  cmp_3/1 -> Bitwise_And3/1
  Bitwise_And3/1 -> tws_3/1, AndN/3, Scope/3
  BS_Req/4 -> cmp_4/1, Scope4/1  "<testSig_Air_bPerTAFSFinalDef>"
  BS_Result/4 -> cmp_4/2, Scope4/2  "<Air_bPerTAFSFinalDef>"
  cmp_4/1 -> Bitwise_And4/1
  Bitwise_And4/1 -> tws_4/1, AndN/4, Scope/4
  BS_Req/5 -> cmp_5/1, Scope5/1  "<testSig_Air_bPerTAFSProvDef>"
  BS_Result/5 -> cmp_5/2, Scope5/2  "<Air_bPerTAFSProvDef>"
  cmp_5/1 -> Bitwise_And5/1
  Bitwise_And5/1 -> tws_5/1, AndN/5, Scope/5
  BS_Req/6 -> cmp_6/1, Scope6/1  "<testSig_Air_facPerCorTAFS>"
  BS_Result/6 -> cmp_6/2, Scope6/2  "<Air_facPerCorTAFS>"
  cmp_6/1 -> Bitwise_And6/1
  Bitwise_And6/1 -> tws_6/1, AndN/6, Scope/6
  BS_Req/7 -> cmp_7/1, Scope7/1  "<testSig_Air_bDtyCycHiDebTAFS_DSM>"
  BS_Result/7 -> cmp_7/2, Scope7/2  "<Air_bDtyCycHiDebTAFS_DSM>"
  cmp_7/1 -> Bitwise_And7/1
  Bitwise_And7/1 -> tws_7/1, AndN/7, Scope/7
  BS_Req/8 -> cmp_8/1, Scope8/1  "<testSig_Air_bDtyCycLoDebTAFS_DSM>"
  BS_Result/8 -> cmp_8/2, Scope8/2  "<Air_bDtyCycLoDebTAFS_DSM>"
  cmp_8/1 -> Bitwise_And8/1
  Bitwise_And8/1 -> tws_8/1, AndN/8, Scope/8
  BS_Req/9 -> cmp_9/1, Scope9/1  "<testSig_Air_bPerHiDebTAFS_DSM>"
  BS_Result/9 -> cmp_9/2, Scope9/2  "<Air_bPerHiDebTAFS_DSM>"
  cmp_9/1 -> Bitwise_And9/1
  Bitwise_And9/1 -> tws_9/1, AndN/9, Scope/9
  BS_Req/10 -> cmp_10/1, Scope10/1  "<testSig_Air_bPerLoDebTAFS_DSM>"
  BS_Result/10 -> cmp_10/2, Scope10/2  "<Air_bPerLoDebTAFS_DSM>"
  cmp_10/1 -> Bitwise_And10/1
  Bitwise_And10/1 -> tws_10/1, AndN/10, Scope/10
  BS_Req/11 -> cmp_11/1, Scope11/1  "<testSig_Air_bVoltTAFSFinalDef>"
  BS_Result/11 -> cmp_11/2, Scope11/2  "<Air_bVoltTAFSFinalDef>"
  cmp_11/1 -> Bitwise_And11/1
  Bitwise_And11/1 -> tws_11/1, AndN/11, Scope/11
  BS_Req/12 -> cmp_12/1, Scope12/1  "<testSig_Air_bVoltTAFSProvDef>"
  BS_Result/12 -> cmp_12/2, Scope12/2  "<Air_bVoltTAFSProvDef>"
  cmp_12/1 -> Bitwise_And12/1
  Bitwise_And12/1 -> tws_12/1, AndN/12, Scope/12
  BS_Req/13 -> cmp_13/1, Scope13/1  "<testSig_Air_bVoltHiDebTAFS_DSM>"
  BS_Result/13 -> cmp_13/2, Scope13/2  "<Air_bVoltHiDebTAFS_DSM>"
  cmp_13/1 -> Bitwise_And13/1
  Bitwise_And13/1 -> tws_13/1, AndN/13, Scope/13
  BS_Req/14 -> cmp_14/1, Scope14/1  "<testSig_Air_bVoltLoDebTAFS_DSM>"
  BS_Result/14 -> cmp_14/2, Scope14/2  "<Air_bVoltLoDebTAFS_DSM>"
  cmp_14/1 -> Bitwise_And14/1
  Bitwise_And14/1 -> tws_14/1, AndN/14, Scope/14
